simulink library "lib_jacobians"  (R2023a)
settings: Solver=VariableStepAuto  StartTime=0.0  StopTime=10.0  RelTol=1e-3
settings Model: Creator=FC_dev1  LastModifiedBy=FC_dev1

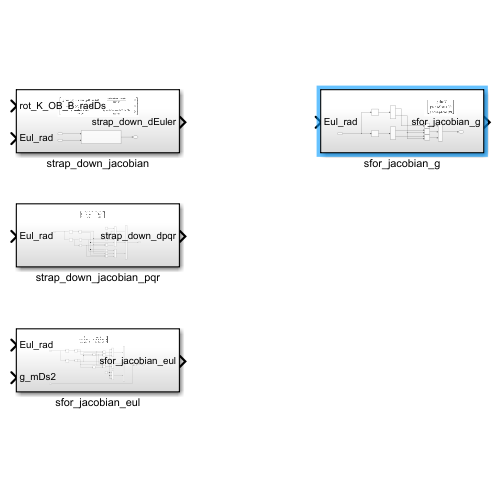
[thumbnail: Simulink's stored preview of the top-level diagram]
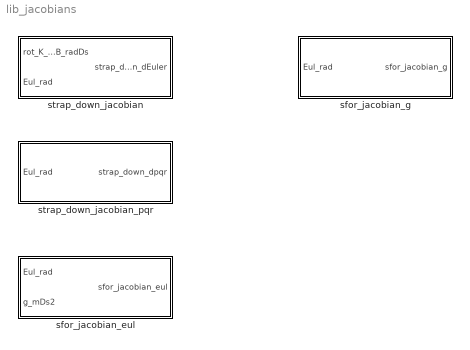
== system lib_jacobians ==
  sfor_jacobian_eul : Subsystem
  sfor_jacobian_g : Subsystem
  strap_down_jacobian : Subsystem
  strap_down_jacobian_pqr : Subsystem

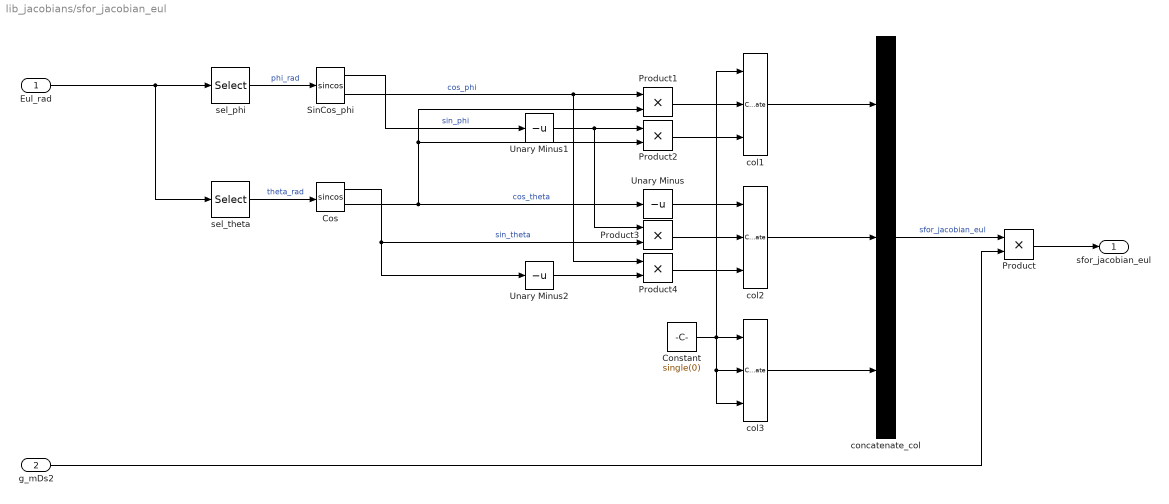
== system lib_jacobians/sfor_jacobian_eul ==
  Eul_rad : Inport  OutDataTypeStr=single  PortDimensions=[3 1]
  g_mDs2 : Inport  Port=2  OutDataTypeStr=single  PortDimensions=1
  Constant : Constant  Value=single(0)
  Cos : Trigonometry  Operator=sincos
  Product{,1..4} (5 alike) : Product
  SinCos_phi : Trigonometry  Operator=sincos
  Unary Minus : UnaryMinus
  Unary Minus1 : UnaryMinus
  Unary Minus2 : UnaryMinus
  col1 : Concatenate  NumInputs=3  Mode=Multidimensional array
  col2 : Concatenate  NumInputs=3  Mode=Multidimensional array
  col3 : Concatenate  NumInputs=3  Mode=Multidimensional array
  concatenate_col : Concatenate  NumInputs=3  Mode=Multidimensional array  ConcatenateDimension=2
  sel_phi : Selector  NumberOfDimensions=2  InputPortWidth=3  IndexOptions=Index vector (dialog),Index vector (dialog)  Indices=1,1  OutputSizes=1,1
  sel_theta : Selector  NumberOfDimensions=2  InputPortWidth=3  IndexOptions=Index vector (dialog),Index vector (dialog)  Indices=2,1  OutputSizes=1,1
  sfor_jacobian_eul : Outport  OutDataTypeStr=single  PortDimensions=[3 3]
  wires:
  Cos/1 -> Unary Minus2/1, Product3/2  "sin_theta"
  SinCos_phi/2 -> Product4/1, Product1/1  "cos_phi"
  SinCos_phi/1 -> Unary Minus1/1  "sin_phi"
  col3/1 -> concatenate_col/3
  col2/1 -> concatenate_col/2
  col1/1 -> concatenate_col/1
  Eul_rad/1 -> sel_theta/1, sel_phi/1
  sel_theta/1 -> Cos/1  "theta_rad"
  concatenate_col/1 -> Product/1  "sfor_jacobian_eul"
  sel_phi/1 -> SinCos_phi/1  "phi_rad"
  Constant/1 -> col1/1, col3/3, col3/2, col3/1
  Product/1 -> sfor_jacobian_eul/1
  g_mDs2/1 -> Product/2
  Product1/1 -> col1/2
  Cos/2 -> Unary Minus/1, Product1/2, Product2/2  "cos_theta"
  Product2/1 -> col1/3
  Unary Minus/1 -> col2/1
  Product3/1 -> col2/2
  Unary Minus1/1 -> Product3/1, Product2/1
  Product4/1 -> col2/3
  Unary Minus2/1 -> Product4/2

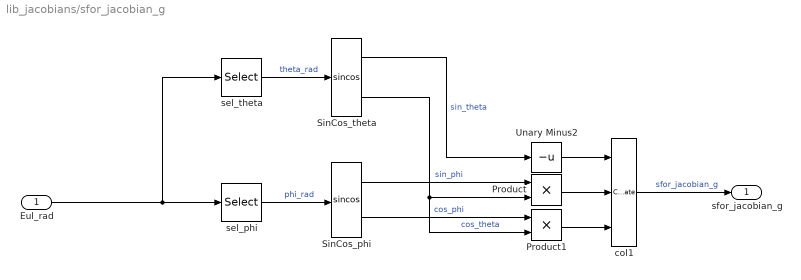
== system lib_jacobians/sfor_jacobian_g ==
  Eul_rad : Inport  OutDataTypeStr=single  PortDimensions=[3 1]
  Product : Product
  Product1 : Product
  SinCos_phi : Trigonometry  Operator=sincos
  SinCos_theta : Trigonometry  Operator=sincos
  Unary Minus2 : UnaryMinus
  col1 : Concatenate  NumInputs=3  Mode=Multidimensional array
  sel_phi : Selector  NumberOfDimensions=2  InputPortWidth=3  IndexOptions=Index vector (dialog),Index vector (dialog)  Indices=1,1  OutputSizes=1,1
  sel_theta : Selector  NumberOfDimensions=2  InputPortWidth=3  IndexOptions=Index vector (dialog),Index vector (dialog)  Indices=2,1  OutputSizes=1,1
  sfor_jacobian_g : Outport  OutDataTypeStr=single  PortDimensions=[3 1]
  wires:
  SinCos_theta/2 -> Product/2, Product1/2  "cos_theta"
  sel_phi/1 -> SinCos_phi/1  "phi_rad"
  col1/1 -> sfor_jacobian_g/1  "sfor_jacobian_g"
  sel_theta/1 -> SinCos_theta/1  "theta_rad"
  Eul_rad/1 -> sel_theta/1, sel_phi/1
  SinCos_phi/1 -> Product/1  "sin_phi"
  SinCos_phi/2 -> Product1/1  "cos_phi"
  SinCos_theta/1 -> Unary Minus2/1  "sin_theta"
  Unary Minus2/1 -> col1/1
  Product/1 -> col1/2
  Product1/1 -> col1/3

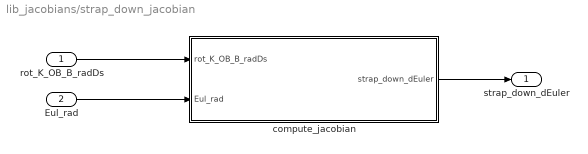
== system lib_jacobians/strap_down_jacobian ==
  rot_K_OB_B_radDs : Inport  OutDataTypeStr=single  PortDimensions=[3 1]
  Eul_rad : Inport  Port=2  OutDataTypeStr=single  PortDimensions=[3 1]
  compute_jacobian : MATLAB Function  TreatAsAtomicUnit=on
  strap_down_dEuler : Outport  OutDataTypeStr=single  PortDimensions=[3 3]
  wires:
  Eul_rad/1 -> compute_jacobian/2(Eul_rad)
  rot_K_OB_B_radDs/1 -> compute_jacobian/1(rot_K_OB_B_radDs)
  compute_jacobian/1(strap_down_dEuler) -> strap_down_dEuler/1

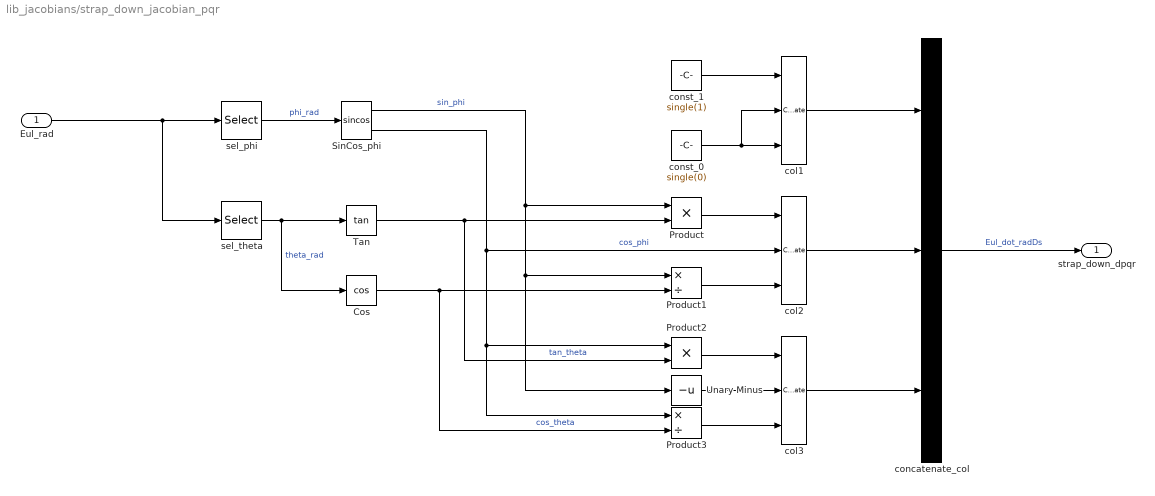
== system lib_jacobians/strap_down_jacobian_pqr ==
  Eul_rad : Inport  OutDataTypeStr=single  PortDimensions=[3 1]
  Cos : Trigonometry  Operator=cos
  Product : Product
  Product1 : Product  Inputs=*/
  Product2 : Product
  Product3 : Product  Inputs=*/
  SinCos_phi : Trigonometry  Operator=sincos
  Tan : Trigonometry  Operator=tan
  Unary Minus : UnaryMinus
  col1 : Concatenate  NumInputs=3  Mode=Multidimensional array
  col2 : Concatenate  NumInputs=3  Mode=Multidimensional array
  col3 : Concatenate  NumInputs=3  Mode=Multidimensional array
  concatenate_col : Concatenate  NumInputs=3  Mode=Multidimensional array  ConcatenateDimension=2
  const_0 : Constant  Value=single(0)
  const_1 : Constant  Value=single(1)
  sel_phi : Selector  NumberOfDimensions=2  InputPortWidth=3  IndexOptions=Index vector (dialog),Index vector (dialog)  Indices=1,1  OutputSizes=1,1
  sel_theta : Selector  NumberOfDimensions=2  InputPortWidth=3  IndexOptions=Index vector (dialog),Index vector (dialog)  Indices=2,1  OutputSizes=1,1
  strap_down_dpqr : Outport  OutDataTypeStr=single  PortDimensions=[3 3]
  wires:
  sel_phi/1 -> SinCos_phi/1  "phi_rad"
  concatenate_col/1 -> strap_down_dpqr/1  "Eul_dot_radDs"
  sel_theta/1 -> Cos/1, Tan/1  "theta_rad"
  Eul_rad/1 -> sel_theta/1, sel_phi/1
  col1/1 -> concatenate_col/1
  col2/1 -> concatenate_col/2
  col3/1 -> concatenate_col/3
  const_1/1 -> col1/1
  const_0/1 -> col1/2, col1/3
  Product/1 -> col2/1
  SinCos_phi/1 -> Unary Minus/1, Product1/1, Product/1  "sin_phi"
  Tan/1 -> Product2/2, Product/2  "tan_theta"
  SinCos_phi/2 -> Product3/1, Product2/1, col2/2  "cos_phi"
  Product1/1 -> col2/3
  Cos/1 -> Product3/2, Product1/2  "cos_theta"
  Product2/1 -> col3/1
  Unary Minus/1 -> col3/2
  Product3/1 -> col3/3

== matlab function lib_jacobians/strap_down_jacobian/compute_jacobian ==
  data: rot_K_OB_B_radDs input single size=[3 1]; strap_down_dEuler output single size=[3 3]; Eul_rad input single size=[3 1]
function strap_down_dEuler = compute_jacobian(rot_K_OB_B_radDs, Eul_rad)

% Initialize output
strap_down_dEuler = zeros(3,3, 'single');

% Auxiliary computations
q_cos_phi = rot_K_OB_B_radDs(2) * cos(Eul_rad(1));
q_sin_phi = rot_K_OB_B_radDs(2) * sin(Eul_rad(1));
r_cos_phi = rot_K_OB_B_radDs(3) * cos(Eul_rad(1));
r_sin_phi = rot_K_OB_B_radDs(3) * sin(Eul_rad(1));
sin_theta = sin(Eul_rad(2));
cos_theta = cos(Eul_rad(2));
% tan_theta = tan(Eul_rad(2));

% Assign non-zero elements
strap_down_dEuler(1) = (q_cos_phi - r_sin_phi)*sin_theta/cos_theta;
strap_down_dEuler(2) = -q_sin_phi - r_cos_phi;
strap_down_dEuler(3) = (q_cos_phi - r_sin_phi)/cos_theta;
strap_down_dEuler(4) = (q_sin_phi + r_cos_phi)/cos_theta^2;
strap_down_dEuler(6) = (q_sin_phi + r_cos_phi)*sin_theta/(cos_theta^2);
